simulink model "Integrated_Model"  (R2020a)
settings: Solver=FixedStepDiscrete  StartTime=0.0  StopTime=10.0  FixedStep=1  RelTol=1e-3
values from neighbouring files (symbols this model uses):
  Ignition : value not decoded    [ALS_Project_dd.sldd]
  Lanes : value not decoded    [ALS_Project_dd.sldd]
  Visual : value not decoded    [ALS_Project_dd.sldd]
undefined symbols (not defined in the file or in its folder): AlsMode, HeadLights, roads
libraries: simulink x29
settings Model: Creator=Pratik shinde  LastModifiedBy=Pratik shinde
settings ConfigComp: DVTestSuiteOptimization=Auto  DVDetectOutOfBounds=on

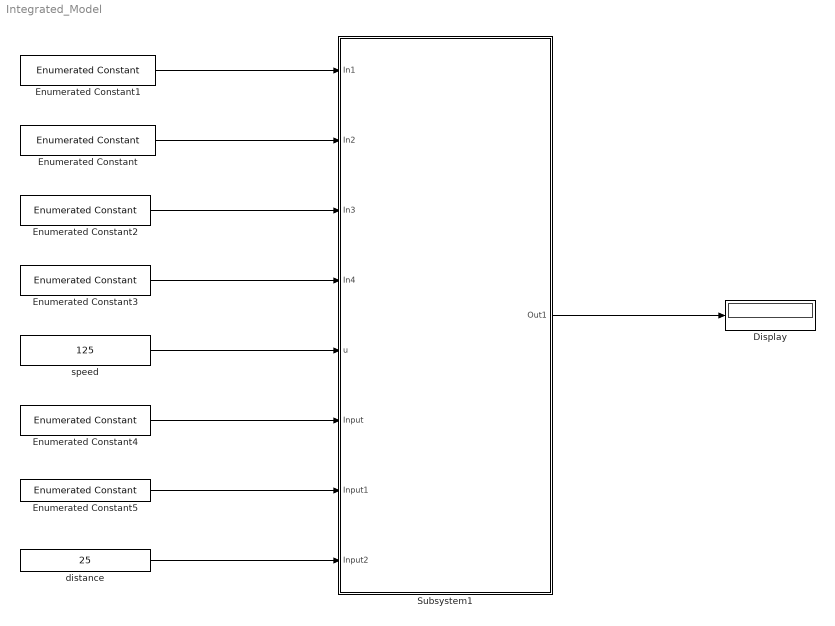
== system Integrated_Model ==
  Display : Display
  Enumerated Constant : simulink/Sources/Enumerated Constant  OutDataTypeStr=Enum: roads  Value=roads.High_way  SampleTime=inf
  Enumerated Constant1 : simulink/Sources/Enumerated Constant  OutDataTypeStr=Enum: AlsMode  Value=AlsMode.On  SampleTime=inf
  Enumerated Constant2 : simulink/Sources/Enumerated Constant  OutDataTypeStr=Enum: Ignition  Value=Ignition.On  SampleTime=inf
  Enumerated Constant3 : simulink/Sources/Enumerated Constant  OutDataTypeStr=Enum: Visual  Value=Visual.Night_Time  SampleTime=inf
  Enumerated Constant4 : simulink/Sources/Enumerated Constant  OutDataTypeStr=Enum: Lanes  Value=Lanes.NoVehicle  SampleTime=inf
  Enumerated Constant5 : simulink/Sources/Enumerated Constant  OutDataTypeStr=Enum: Lanes  Value=Lanes.Lane1_left  SampleTime=inf
  Subsystem1 : Subsystem
  distance : Constant  Value=25
  speed : Constant  Value=125
  wires:
  Enumerated Constant2/1 -> Subsystem1/3(In3)
  Subsystem1/1(Out1) -> Display/1
  Enumerated Constant1/1 -> Subsystem1/1(In1)
  Enumerated Constant5/1 -> Subsystem1/7(Input1)
  distance/1 -> Subsystem1/8(Input2)
  Enumerated Constant/1 -> Subsystem1/2(In2)
  Enumerated Constant3/1 -> Subsystem1/4(In4)
  speed/1 -> Subsystem1/5(u)
  Enumerated Constant4/1 -> Subsystem1/6(Input)

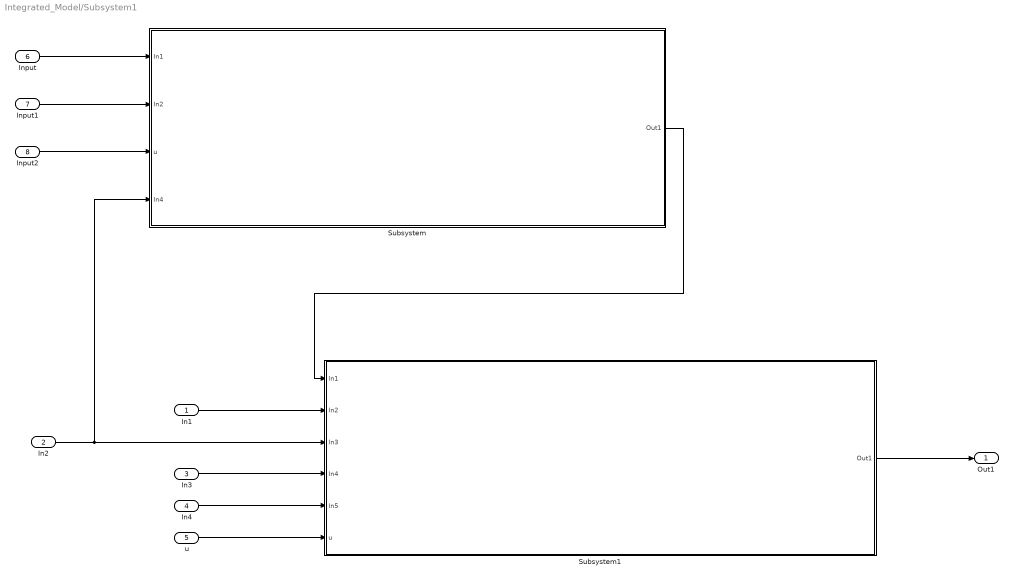
== system Integrated_Model/Subsystem1 ==
  In1 : Inport
  In2 : Inport  Port=2
  In3 : Inport  Port=3
  In4 : Inport  Port=4
  u : Inport  Port=5
  Input : Inport  Port=6
  Input1 : Inport  Port=7
  Input2 : Inport  Port=8
  Subsystem : Subsystem
  Subsystem1 : Subsystem
  Out1 : Outport
  wires:
  Input/1 -> Subsystem/1(In1)
  Input1/1 -> Subsystem/2(In2)
  Input2/1 -> Subsystem/3(u)
  In3/1 -> Subsystem1/4(In4)
  In4/1 -> Subsystem1/5(In5)
  u/1 -> Subsystem1/6(u)
  Subsystem/1(Out1) -> Subsystem1/1(In1)
  In1/1 -> Subsystem1/2(In2)
  In2/1 -> Subsystem/4(In4), Subsystem1/3(In3)
  Subsystem1/1(Out1) -> Out1/1

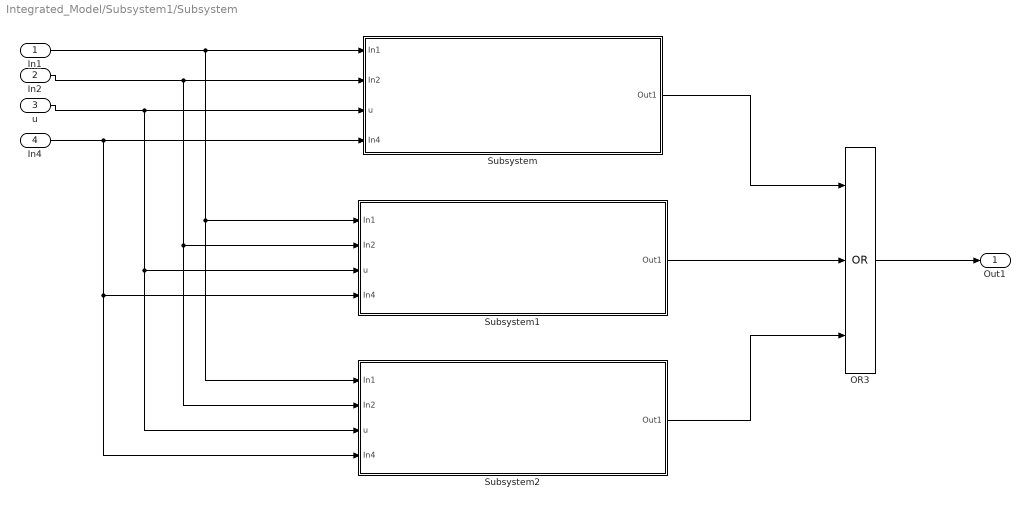
== system Integrated_Model/Subsystem1/Subsystem ==
  In1 : Inport
  In2 : Inport  Port=2
  u : Inport  Port=3
  In4 : Inport  Port=4
  OR3 : Logic  Operator=OR  Inputs=3  AllPortsSameDT=off  OutDataTypeStr=boolean
  Subsystem : Subsystem
  Subsystem1 : Subsystem
  Subsystem2 : Subsystem
  Out1 : Outport
  wires:
  In4/1 -> Subsystem2/4(In4), Subsystem1/4(In4), Subsystem/4(In4)
  Subsystem1/1(Out1) -> OR3/2
  Subsystem/1(Out1) -> OR3/1
  Subsystem2/1(Out1) -> OR3/3
  In2/1 -> Subsystem2/2(In2), Subsystem1/2(In2), Subsystem/2(In2)
  u/1 -> Subsystem2/3(u), Subsystem1/3(u), Subsystem/3(u)
  In1/1 -> Subsystem2/1(In1), Subsystem1/1(In1), Subsystem/1(In1)
  OR3/1 -> Out1/1

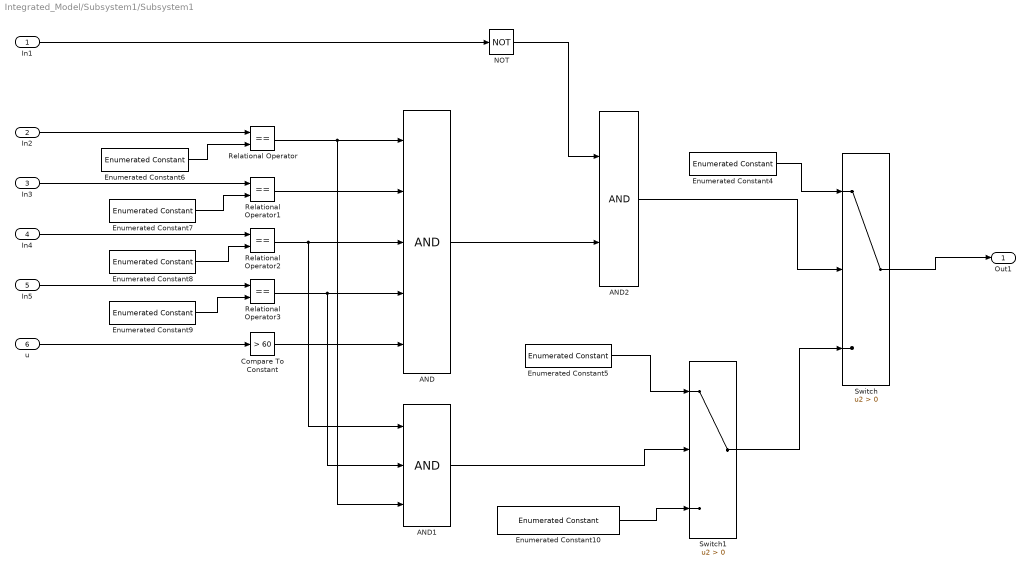
== system Integrated_Model/Subsystem1/Subsystem1 ==
  In1 : Inport
  In2 : Inport  Port=2
  In3 : Inport  Port=3
  In4 : Inport  Port=4
  In5 : Inport  Port=5
  u : Inport  Port=6
  AND : Logic  Inputs=5  AllPortsSameDT=off  OutDataTypeStr=boolean
  AND1 : Logic  Inputs=3  AllPortsSameDT=off  OutDataTypeStr=boolean
  AND2 : Logic  AllPortsSameDT=off  OutDataTypeStr=boolean
  Compare To Constant : simulink/Logic and Bit Operations/Compare To Constant  relop=>  const=60  OutDataTypeStr=boolean
  Enumerated Constant10 : simulink/Sources/Enumerated Constant  OutDataTypeStr=Enum:HeadLights  Value=HeadLights.HeadLight_Off  SampleTime=inf
  Enumerated Constant4 : simulink/Sources/Enumerated Constant  OutDataTypeStr=Enum: HeadLights  Value=HeadLights.HighBeam  SampleTime=inf
  Enumerated Constant5 : simulink/Sources/Enumerated Constant  OutDataTypeStr=Enum: HeadLights  Value=HeadLights.LowBeam  SampleTime=inf
  Enumerated Constant6 : simulink/Sources/Enumerated Constant  OutDataTypeStr=Enum: AlsMode  Value=AlsMode.On  SampleTime=inf
  Enumerated Constant7 : simulink/Sources/Enumerated Constant  OutDataTypeStr=Enum: roads  Value=roads.High_way  SampleTime=inf
  Enumerated Constant8 : simulink/Sources/Enumerated Constant  OutDataTypeStr=Enum: Ignition  Value=Ignition.On  SampleTime=inf
  Enumerated Constant9 : simulink/Sources/Enumerated Constant  OutDataTypeStr=Enum: Visual  Value=Visual.Night_Time  SampleTime=inf
  NOT : Logic  Operator=NOT  IconShape=distinctive  AllPortsSameDT=off  OutDataTypeStr=boolean
  Relational Operator{,1..3} (4 alike) : RelationalOperator  Operator===  OutDataTypeStr=boolean  RndMeth=Simplest
  Switch : Switch  Criteria=u2 > Threshold
  Switch1 : Switch  Criteria=u2 > Threshold
  Out1 : Outport
  wires:
  Relational Operator3/1 -> AND1/2, AND/4
  Relational Operator/1 -> AND1/3, AND/1
  Relational Operator2/1 -> AND1/1, AND/3
  Enumerated Constant7/1 -> Relational Operator1/2
  Switch1/1 -> Switch/3
  Enumerated Constant10/1 -> Switch1/3
  AND1/1 -> Switch1/2
  Enumerated Constant9/1 -> Relational Operator3/2
  u/1 -> Compare To Constant/1
  Compare To Constant/1 -> AND/5
  In2/1 -> Relational Operator/1
  In3/1 -> Relational Operator1/1
  AND/1 -> AND2/2
  Enumerated Constant8/1 -> Relational Operator2/2
  Enumerated Constant5/1 -> Switch1/1
  In4/1 -> Relational Operator2/1
  Switch/1 -> Out1/1
  Relational Operator1/1 -> AND/2
  In5/1 -> Relational Operator3/1
  Enumerated Constant4/1 -> Switch/1
  In1/1 -> NOT/1
  Enumerated Constant6/1 -> Relational Operator/2
  NOT/1 -> AND2/1
  AND2/1 -> Switch/2

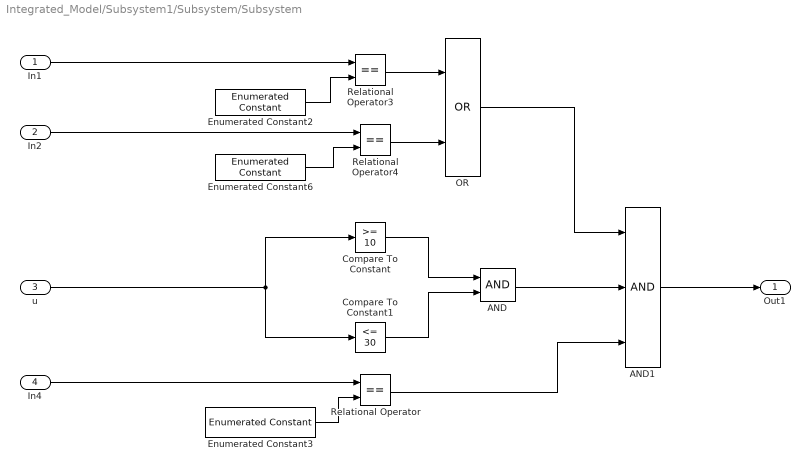
== system Integrated_Model/Subsystem1/Subsystem/Subsystem ==
  In1 : Inport
  In2 : Inport  Port=2
  u : Inport  Port=3
  In4 : Inport  Port=4
  AND : Logic  AllPortsSameDT=off  OutDataTypeStr=boolean
  AND1 : Logic  Inputs=3  AllPortsSameDT=off  OutDataTypeStr=boolean
  Compare To Constant : simulink/Logic and Bit Operations/Compare To Constant  relop=>=  const=10  OutDataTypeStr=boolean
  Compare To Constant1 : simulink/Logic and Bit Operations/Compare To Constant  relop=<=  const=30  OutDataTypeStr=boolean
  Enumerated Constant2 : simulink/Sources/Enumerated Constant  OutDataTypeStr=Enum: Lanes  Value=Lanes.Lane1_right  SampleTime=inf
  Enumerated Constant3 : simulink/Sources/Enumerated Constant  OutDataTypeStr=Enum: roads  Value=roads.High_way  SampleTime=inf
  Enumerated Constant6 : simulink/Sources/Enumerated Constant  OutDataTypeStr=Enum: Lanes  Value=Lanes.Lane1_left  SampleTime=inf
  OR : Logic  Operator=OR  AllPortsSameDT=off  OutDataTypeStr=boolean
  Relational Operator : RelationalOperator  Operator===  OutDataTypeStr=boolean  RndMeth=Simplest
  Relational Operator3 : RelationalOperator  Operator===  OutDataTypeStr=boolean  RndMeth=Simplest
  Relational Operator4 : RelationalOperator  Operator===  OutDataTypeStr=boolean  RndMeth=Simplest
  Out1 : Outport
  wires:
  Enumerated Constant6/1 -> Relational Operator4/2
  Relational Operator3/1 -> OR/1
  Compare To Constant/1 -> AND/1
  OR/1 -> AND1/1
  u/1 -> Compare To Constant/1, Compare To Constant1/1
  Relational Operator/1 -> AND1/3
  In4/1 -> Relational Operator/1
  Enumerated Constant2/1 -> Relational Operator3/2
  In2/1 -> Relational Operator4/1
  Enumerated Constant3/1 -> Relational Operator/2
  AND/1 -> AND1/2
  Compare To Constant1/1 -> AND/2
  Relational Operator4/1 -> OR/2
  In1/1 -> Relational Operator3/1
  AND1/1 -> Out1/1

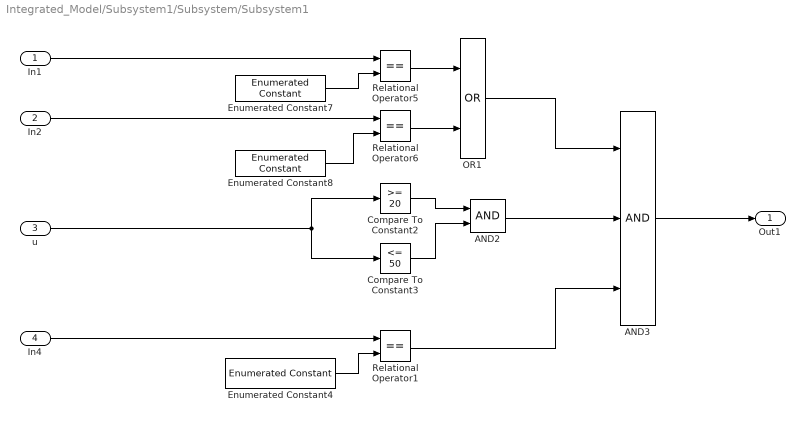
== system Integrated_Model/Subsystem1/Subsystem/Subsystem1 ==
  In1 : Inport
  In2 : Inport  Port=2
  u : Inport  Port=3
  In4 : Inport  Port=4
  AND2 : Logic  AllPortsSameDT=off  OutDataTypeStr=boolean
  AND3 : Logic  Inputs=3  AllPortsSameDT=off  OutDataTypeStr=boolean
  Compare To Constant2 : simulink/Logic and Bit Operations/Compare To Constant  relop=>=  const=20  OutDataTypeStr=boolean
  Compare To Constant3 : simulink/Logic and Bit Operations/Compare To Constant  relop=<=  const=50  OutDataTypeStr=boolean
  Enumerated Constant4 : simulink/Sources/Enumerated Constant  OutDataTypeStr=Enum: roads  Value=roads.High_way  SampleTime=inf
  Enumerated Constant7 : simulink/Sources/Enumerated Constant  OutDataTypeStr=Enum: Lanes  Value=Lanes.Lane2_right  SampleTime=inf
  Enumerated Constant8 : simulink/Sources/Enumerated Constant  OutDataTypeStr=Enum: Lanes  Value=Lanes.Lane2_left  SampleTime=inf
  OR1 : Logic  Operator=OR  AllPortsSameDT=off  OutDataTypeStr=boolean
  Relational Operator1 : RelationalOperator  Operator===  OutDataTypeStr=boolean  RndMeth=Simplest
  Relational Operator5 : RelationalOperator  Operator===  OutDataTypeStr=boolean  RndMeth=Simplest
  Relational Operator6 : RelationalOperator  Operator===  OutDataTypeStr=boolean  RndMeth=Simplest
  Out1 : Outport
  wires:
  u/1 -> Compare To Constant2/1, Compare To Constant3/1
  AND3/1 -> Out1/1
  In2/1 -> Relational Operator6/1
  Enumerated Constant4/1 -> Relational Operator1/2
  Relational Operator1/1 -> AND3/3
  Compare To Constant3/1 -> AND2/2
  Enumerated Constant7/1 -> Relational Operator5/2
  OR1/1 -> AND3/1
  Compare To Constant2/1 -> AND2/1
  AND2/1 -> AND3/2
  In4/1 -> Relational Operator1/1
  Enumerated Constant8/1 -> Relational Operator6/2
  Relational Operator6/1 -> OR1/2
  Relational Operator5/1 -> OR1/1
  In1/1 -> Relational Operator5/1

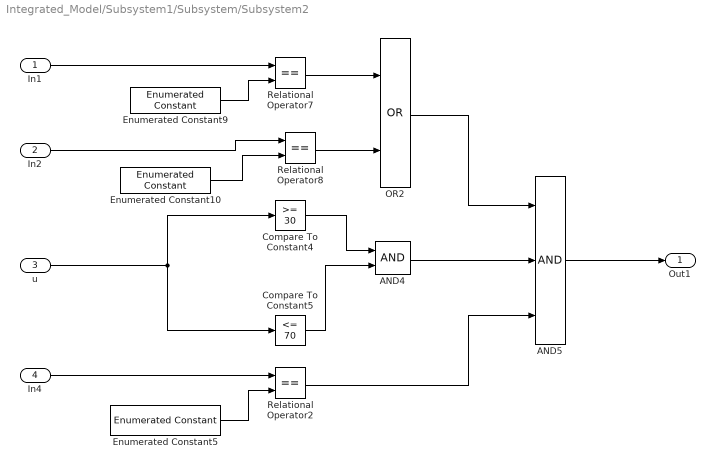
== system Integrated_Model/Subsystem1/Subsystem/Subsystem2 ==
  In1 : Inport
  In2 : Inport  Port=2
  u : Inport  Port=3
  In4 : Inport  Port=4
  AND4 : Logic  AllPortsSameDT=off  OutDataTypeStr=boolean
  AND5 : Logic  Inputs=3  AllPortsSameDT=off  OutDataTypeStr=boolean
  Compare To Constant4 : simulink/Logic and Bit Operations/Compare To Constant  relop=>=  const=30  OutDataTypeStr=boolean
  Compare To Constant5 : simulink/Logic and Bit Operations/Compare To Constant  relop=<=  const=70  OutDataTypeStr=boolean
  Enumerated Constant10 : simulink/Sources/Enumerated Constant  OutDataTypeStr=Enum: Lanes  Value=Lanes.Lane3_left  SampleTime=inf
  Enumerated Constant5 : simulink/Sources/Enumerated Constant  OutDataTypeStr=Enum: roads  Value=roads.High_way  SampleTime=inf
  Enumerated Constant9 : simulink/Sources/Enumerated Constant  OutDataTypeStr=Enum: Lanes  Value=Lanes.Lane3_right  SampleTime=inf
  OR2 : Logic  Operator=OR  AllPortsSameDT=off  OutDataTypeStr=boolean
  Relational Operator2 : RelationalOperator  Operator===  OutDataTypeStr=boolean  RndMeth=Simplest
  Relational Operator7 : RelationalOperator  Operator===  OutDataTypeStr=boolean  RndMeth=Simplest
  Relational Operator8 : RelationalOperator  Operator===  OutDataTypeStr=boolean  RndMeth=Simplest
  Out1 : Outport
  wires:
  u/1 -> Compare To Constant4/1, Compare To Constant5/1
  Relational Operator8/1 -> OR2/2
  AND5/1 -> Out1/1
  In4/1 -> Relational Operator2/1
  Relational Operator7/1 -> OR2/1
  Compare To Constant5/1 -> AND4/2
  Relational Operator2/1 -> AND5/3
  OR2/1 -> AND5/1
  Enumerated Constant5/1 -> Relational Operator2/2
  Compare To Constant4/1 -> AND4/1
  AND4/1 -> AND5/2
  Enumerated Constant9/1 -> Relational Operator7/2
  Enumerated Constant10/1 -> Relational Operator8/2
  In2/1 -> Relational Operator8/1
  In1/1 -> Relational Operator7/1
